simulink model "EKF_sim"  (R2020a)
settings: Solver=VariableStepAuto  StartTime=0.0  StopTime=257  RelTol=1e-3
values from neighbouring files (symbols this model uses):
  acc_variance = 4.8e-2    (= 0.048)    [init.m]
  bias_acc_variance = 4e-14    [init.m]
  bias_gyro_variance = 4e-14    [init.m]
  Delta2 = [260.168 -23.8158 1.64305]    [init.m]
  DT = EKF_DT    (= 0.01)    [init.m]
  EKF_DT = 0.01    [init.m]
  g = 9.81    [init.m]
  GPS_variance = 5    [init.m]
  gyro_variance = 4.8e-6    (= 4.8e-06)    [init.m]
  h0 = 38.8887000000000000    (= 38.8887)    [init.m]
  head_variance = 5e-2    (= 0.05)    [init.m]
  init_time = 4    [init.m]
  lambda_xa = 1e-4    (= 0.0001)    [init.m]
  lambda_xg = 1e-3    (= 0.001)    [init.m]
  lat0 = 36.7144590750000006    (= 36.714459075)    [init.m]
  lon0 = -4.4789588283333330    (= -4.47895882833)    [init.m]
  SHOE_buffer_N = 100    [init.m]
  SHOE_threshold = 2000    [init.m]
  t1_end = 100    [init.m]
  t1_start = 90    [init.m]
  t2_end = 193    [init.m]
  t2_start = 183    [init.m]
  t3_end = 213    [init.m]
  t3_start = 203    [init.m]
  t4_end = 244    [init.m]
  t4_start = 237    [init.m]
  type_of_GPS = 1    [init.m]
  vel_variance = 1e-2    (= 0.01)    [init.m]
  zero_vel_period = 0.1    [init.m]
(part 3 of 5)

== matlab function EKF_sim/EKF_nb/System Update/Flag Update/flag_updates ==
  data: time input; flag_updates_vector output size=1 3; SHOE_idx output; SHOE_buffer output; clk_zero_vel input; gyro input; acc input; pos_GPS input; hea_GPS input; SHOE_idx_prec input; SHOE_buffer_prec input; GPS_prec input; g parameter; GPS output; acc_variance parameter; gyro_variance parameter; SHOE_threshold parameter; SHOE_buffer_N parameter; t1_start parameter; t1_end parameter; t2_start parameter; t2_end parameter; t3_start parameter; t3_end parameter; ris output; t4_start parameter; t4_end parameter
% --------------------        flag_updates          -------------------- %
%{
% This function generate a flag vector containing informations of updates 
% for the correction step. There are three types of updates:

%  1. Zero Velocity constraints: we assume the vehicle moves only along its
%     x body axis direction, so the velocity in y and z axis are assumed to
%     be equal to zero.
%     The frequency of this update is based on signal 'clk_zero_vel', based
%     on 'zero_vel_period' parameter.
  
%  2. No-accelerating mode: when we detect a very low acceleration of the
%     vehicle, we can assume the accelerometer measures the gravity vector.
%     In this case we can update roll and pitch angles. SHOE algorithm is
%     used to detect a no-accelerating situation. (see [23] I. Skog et al., 
%     “Zero-Velocity Detection An Algorithm Evaluation,” IEEE Transactions 
%     on Biomedical Engineering, vol.57, no.11, pp.2657-2666, November
%     2010.)

%  3. Position and Heading updates: when a new value from GPS is detected,
%     position and heading is updated.

% In order to evaluate the EKF with GPS outages, we can block position and
% headings correction forced the corresponding flag to zero. This happens 
% in time intervals defined by the parameters t*_start and t*_end.

% Input:
%   time             : simulation time
%   clk_zero_vel     : clock of zero velocity constraints update
%   gyro             : [3x1] gyroscope measurement
%   acc              : [3x1] accelerometer measurement
%   pos_GPS          : [3x1] GPS data in NED
%   hea_GPS          : [1] Heading value from GPS data
%   SHOE_idx_prec    : previous buffer index for computation of SHOE algorithm
%   SHOE_buffer_prec : previous buffer for computation of SHOE algorithm
%   GPS_prec         : [4x1] previous data from GPS
%   g                : gravity acceleration
%   acc_variance     : Accelerometer Variance
%   gyro_variance    : Gyroscope Variance
%   SHOE_threshold   : Threshold for SHOE algorithm
%   SHOE_buffer_N    : Dimension of buffer for SHOE algorithm
%   t*_start         : start time i for GPS outage
%   t*_end           : end time i for GPS outage

% Output:
%   flag_updates_vector : [3x1] flag vector for new updates
%   SHOE_idx            : buffer index for computation of SHOE algorithm
%   SHOE_buffer         : buffer for computation of SHOE algorithm
%   GPS                 : [4x1] data from GPS
%   ris                 : Resultimg value of SHOE algorithm 
%}
%%
function [flag_updates_vector, SHOE_idx, SHOE_buffer, GPS,ris]  = flag_updates(time,clk_zero_vel, gyro, acc, pos_GPS, hea_GPS,...
                                                                         SHOE_idx_prec, SHOE_buffer_prec, GPS_prec, ...
                                                                         g, acc_variance, gyro_variance, SHOE_threshold, SHOE_buffer_N,...
                                                                         t1_start,t1_end,t2_start,t2_end,t3_start,t3_end,t4_start,t4_end)
    flag_updates_vector = zeros(1,3);
    
    %Dynamical constraints update (zero velocity)
    if clk_zero_vel == 1
        flag_updates_vector(1) = 1;
    end
    
    %Roll and Pitch Updates
    [SHOE_buffer, SHOE_idx, SHOE_flag,ris] = SHOE_detector(gyro, acc, SHOE_buffer_prec, SHOE_idx_prec, ...
                                                            SHOE_buffer_N, acc_variance, gyro_variance, SHOE_threshold, g); 
    if SHOE_flag == 1
        flag_updates_vector(2) = 1;
    end

    %Position and Heading Updates
    GPS = [pos_GPS(1), pos_GPS(2), pos_GPS(3), hea_GPS]';

    if ~isequal(GPS,GPS_prec)
        flag_updates_vector(3) = 1;
    end
    
    %Forced GPS outages
    if time > t1_start && time < t1_end
        flag_updates_vector(3) = 0;
    end
    if time > t2_start && time < t2_end
        flag_updates_vector(3) = 0;
    end
    if time > t3_start && time < t3_end
        flag_updates_vector(3) = 0;
    end
    if time > t4_start && time < t4_end
        flag_updates_vector(3) = 0;
    end
end

%% SHOE detector (ref.[23])
% This function detects if the acceleration of the vehicle is nearly zero.
% In that case we use the accelerometer measurements to estimates the 
% gravity vector in body frame and use it to update roll and pitch.
% For this purpose the mean of the last N measurements of accelerometer are
% compared to the gravity vector (magnitide and direction) and we use 
% gyroscope measurement to check if the vehicle is rotating. The resulting
% value stored in [ris] is compared with the SHOE Threshold.

function [SHOE_buffer, SHOE_idx, SHOE_flag,ris] = SHOE_detector(gyro, acc, SHOE_buffer, SHOE_idx, ...
                                                            SHOE_buffer_N, acc_variance, gyro_variance, SHOE_threshold, g) 
    %Buffer update with new measurement
    SHOE_buffer(SHOE_idx,:) = [acc(1), acc(2), acc(3), gyro(1), gyro(2), gyro(3)];
    SHOE_idx = SHOE_idx + 1;
    if SHOE_idx > SHOE_buffer_N
        SHOE_idx = 1;
    end

    %Detector Algorithm
    ya_n = [0 0 0];
    for i = 1:SHOE_buffer_N
        ya_n = ya_n + SHOE_buffer(i,1:3);	
    end
    ya_n = ya_n/SHOE_buffer_N;
    
    %calculate resulting maen value
    ris = 0; 
    for i = 1:SHOE_buffer_N
        ris = ris + (1/(acc_variance))*((norm(SHOE_buffer(i,1:3) - g*ya_n/norm(ya_n)))^2) + ...
                  + (1/(gyro_variance))*((norm(SHOE_buffer(i,4:6)))^2);
    end
    ris = ris/SHOE_buffer_N;
    
    if ris < SHOE_threshold
        SHOE_flag = 1;
    else 
        SHOE_flag = 0;
    end
end

%% %%%%%%%%%%%%%%%%%%%%%%%%%%%%%%%%%%%%%%%%%%%%%%%%%%%%%%%%%%%%%%%%%%%%%%%
     %%%%%%%%% Direct EKF for 6D Pose,  Marco Borraccino %%%%%%%%%%
     %%%%%%%%%   SGN Project, University of Pisa, 2021   %%%%%%%%%%
%%%%%%%%%%%%%%%%%%%%%%%%%%%%%%%%%%%%%%%%%%%%%%%%%%%%%%%%%%%%%%%%%%%%%%%%%%

== matlab function EKF_sim/EKF_nb/System Update/correction_step ==
  data: x_k_1 input; x_k output; P_k_1 input; e input size=9 1; H input size=9 16; R_k input size=9 9; P_k output; flag_init input
% --------------------         correction           -------------------- %
%{
% This function computes the correction step of the Kalman Filter. When new
% updates are avaiable, the Kalman Gain is updated and the vector state and
% matrix P too.

% Input:
%     x_k_1     : [16x1] state vector before correction step
%     P_k_1     : [16x16] matrix P before correction step
%     e         : [] Error between current measure and predicted measure
%     H         : [] Jacobian of prediction model measurement with respect 
%                 to state x
%     R_k       : [] Measurement Noise Covariance Matrix at time k
%     flag_init : flag for initialization task

% Output:
%     x_k       : [16x1] state vector after correction step
%     P_k       : [16x16] matrix P after correction step

% The formulas are?
%     S_k = H*P_k_1*H' + R_k;
%     K_k = P_k_1*H'*(inv(S_k));
%     P_k = (eye(16)-(K_k*H))*P_k_1;         
%     x_k = x_k_1 + K_k * e;
%}
%%
function [x_k, P_k] = correction(x_k_1, P_k_1, ...
                                 e, H, R_k, flag_init)
     x_k = zeros(16,1);
     P_k = zeros(16,16);
     
     if flag_init ~= -1
                
          S_k = H*P_k_1*H' + R_k;
          K_k = P_k_1*H'*(inv(S_k));

          P_k = (eye(16)-(K_k*H))*P_k_1;         
          x_k = x_k_1 + K_k * e;
     end
end

%% %%%%%%%%%%%%%%%%%%%%%%%%%%%%%%%%%%%%%%%%%%%%%%%%%%%%%%%%%%%%%%%%%%%%%%%
     %%%%%%%%% Direct EKF for 6D Pose,  Marco Borraccino %%%%%%%%%%
     %%%%%%%%%   SGN Project, University of Pisa, 2021   %%%%%%%%%%
%%%%%%%%%%%%%%%%%%%%%%%%%%%%%%%%%%%%%%%%%%%%%%%%%%%%%%%%%%%%%%%%%%%%%%%%%%

== matlab function EKF_sim/EKF_nb/System Update/virtual ==
  data: x_k input; R_ input; e output size=9 1; H output size=9 16; R_k output size=9 9; flag_updates_vector input; acc input; pos_GPS input; hea_GPS input; g parameter
% --------------------          virtual            -------------------- %
%{
% This function check the flag_updates_vector and produces the terms 'e',
% 'H' and 'R' based on it. When a flag update is set to zero by the
% previous function 'virtual', the dimensions of vector 'e' and matrices 
% 'H' and 'R' change to avoid wrong correction.
% There are three types of updates:

%  1. Zero Velocity constraints: we assume the vehicle moves only along its
%     x body axis direction, so the velocity in y and z axis are assumed to
%     be equal to zero.

%  2. No-accelerating mode: when we detect a very low acceleration of the
%     vehicle, we can assume the accelerometer measures the gravity vector.
%     In this case we can update roll and pitch angles.

%  3. Position and Heading updates: when a new value from GPS is detected,
%     position and heading is updated.

% For more deatils about matrix 'H' and the change of dimension, see file
% 'calcolo_matrice_H' and 'cutter_matrix'.

% Input:
%     x_k                 : [16x1] state vector before correction step
%     R_                  : [9x9] Measurement Noise Covariance Matrix
%     flag_updates_vector : [3x1] flag vector for new updates
%     acc                 : [3x1] Accelerometer Measurement
%     pos_GPS             : [3x1] GPS data in NED
%     hea_GPS             : [1] Heading value from GPS data
%     g                   : gravity acceleration

% Output:
%     e         : [] Error between current measure and predicted measure
%     H         : [] Jacobian of prediction model measurement with respect  
%                 to state x
%     R_k       : [] Measurement Noise Covariance Matrix at time k
%}
%%
function [e, H, R_k] = virtual(x_k, R_, flag_updates_vector, acc, pos_GPS, hea_GPS, g)

    e = zeros(9,1);
    h = zeros(9,1);
    z = zeros(9,1);
    H = zeros(9,16);
    q = x_k(1:4);
    
    %Dynamical constraints update (zero velocity)
    if  flag_updates_vector(1) == 1
        %hv0 = zeros(3,1);
        v  = x_k(11:13);
        Rnb = fromq2rot(q(1),q(2),q(3),q(4));
        hv0 = Rnb'*v;
        
        %z = z + [0       0    0 0 0 0 0 0 0]';
        h = h + [hv0(2) hv0(3) 0 0 0 0 0 0 0]';
        
        [H(1,:), H(2,:)]= calcolo_Hv0(q(1),q(2),q(3),q(4),v(1),v(2),v(3));
    end
    
    %Roll and Pitch Updates    
    if flag_updates_vector(2) == 1
        %hg = zeros(3,1);
        Rnb = fromq2rot(q(1),q(2),q(3),q(4));
        hg = Rnb'*[0 0 -g]';
        
        z = z + [0 0 acc(1) acc(2) acc(3) 0 0 0 0]';
        h = h + [0 0  hg(1)  hg(2)  hg(3) 0 0 0 0]';
        
        [H(3,:), H(4,:), H(5,:)]= calcolo_Hg(q(1),q(2),q(3),q(4),g);

    end
    
    %Position and Heading Updates
    if flag_updates_vector(3) == 1
        
        r = x_k(8:10);
        htheta = atan2(2*(q(2)*q(3)-q(1)*q(4)), 1-2*(q(3)^2+q(4)^2));
        
        z = z + [0 0 0 0 0 pos_GPS(1) pos_GPS(2) pos_GPS(3) hea_GPS]';
        h = h + [0 0 0 0 0    r(1)       r(2)       r(3)    htheta ]';
 
        H(6,:) = [0, 0, 0, 0, 0, 0, 0, 1, 0, 0, 0, 0, 0, 0, 0, 0];
        H(7,:) = [0, 0, 0, 0, 0, 0, 0, 0, 1, 0, 0, 0, 0, 0, 0, 0];
        H(8,:) = [0, 0, 0, 0, 0, 0, 0, 0, 0, 1, 0, 0, 0, 0, 0, 0];
        H(9,:)= calcolo_Htheta(q(1),q(2),q(3),q(4));  
    end
    e = z - h;
    coder.extrinsic('wrapToPi');
    if e(9)> pi
        e(9) = wrapToPi(e(9));
    end
    
    %After the generation of 'e', 'H' and 'R', we eliminate row and columns
    %of them if they are not used. The resultanting scaled vector and 
    %matrix are used in the next correction step function.
    R=R_;
    i=0;
    if  flag_updates_vector(1) == 0
        H(1-i,:) = [];
        e(1-i) = [];
        R(1-i,:) = [];
        R(:,1-i) = [];
        i=i+1;
        H(2-i,:) = [];
        e(2-i) = [];
        R(2-i,:) = [];
        R(:,2-i) = [];
        i=i+1;
    end
    if  flag_updates_vector(2) == 0
        H(3-i,:) = [];
        e(3-i) = [];
        R(3-i,:) = [];
        R(:,3-i) = [];
        i=i+1;
        H(4-i,:) = [];
        e(4-i) = [];
        R(4-i,:) = [];
        R(:,4-i) = [];
        i=i+1;
        H(5-i,:) = [];
        e(5-i) = [];
        R(5-i,:) = [];
        R(:,5-i) = [];
        i=i+1;
    end
    if  flag_updates_vector(3) == 0
        H(6-i,:) = [];
        e(6-i) = [];
        R(6-i,:) = [];
        R(:,6-i) = [];
        i=i+1;
        H(7-i,:) = [];
        e(7-i) = [];
        R(7-i,:) = [];
        R(:,7-i) = [];
        i=i+1;
        H(8-i,:) = [];
        e(8-i) = [];
        R(8-i,:) = [];
        R(:,8-i) = [];
        i=i+1;
        H(9-i,:) = [];
        e(9-i) = [];
        R(9-i,:) = [];
        R(:,9-i) = [];
    end
    R_k=R;
end

%% Auxiliary Functions
% This function computes the rotation matrix from quaternion
function rot = fromq2rot(q1,q2,q3,q4)
    rot = [q1^2+q2^2-q3^2-q4^2, 2*(q2*q3-q1*q4), 2*(q1*q3+q2*q4); ...
           2*(q2*q3+q1*q4), q1^2-q2^2+q3^2-q4^2, 2*(q3*q4-q1*q2); ...
           2*(q2*q4-q1*q3), 2*(q1*q2+q3*q4), q1^2-q2^2-q3^2+q4^2];
end
%%
% These functions calculate the H matrix elements
% See 'calcolo_matrice_H_nb.m' for the symbolic calculation used
function [Hv01 , Hv02] = calcolo_Hv0(q1,q2,q3,q4,vx,vy,vz)  
    Hv01 = [ 2*q1*vy - 2*q4*vx + 2*q2*vz, 2*q3*vx - 2*q2*vy + 2*q1*vz, 2*q2*vx + 2*q3*vy + 2*q4*vz, 2*q3*vz - 2*q4*vy - 2*q1*vx, 0, 0, 0, 0, 0, 0, 2*q2*q3 - 2*q1*q4, q1^2 - q2^2 + q3^2 - q4^2, 2*q1*q2 + 2*q3*q4, 0, 0, 0];
    Hv02 = [ 2*q3*vx - 2*q2*vy + 2*q1*vz, 2*q4*vx - 2*q1*vy - 2*q2*vz, 2*q1*vx + 2*q4*vy - 2*q3*vz, 2*q2*vx + 2*q3*vy + 2*q4*vz, 0, 0, 0, 0, 0, 0, 2*q1*q3 + 2*q2*q4, 2*q3*q4 - 2*q1*q2, q1^2 - q2^2 - q3^2 + q4^2, 0, 0, 0];
end
function [Hg1 , Hg2, Hg3] = calcolo_Hg(q1,q2,q3,q4,g)
    Hg1 = [  2*g*q3, -2*g*q4,  2*g*q1, -2*g*q2, 0, 0, 0, 0, 0, 0, 0, 0, 0, 0, 0, 0];
    Hg2 = [ -2*g*q2, -2*g*q1, -2*g*q4, -2*g*q3, 0, 0, 0, 0, 0, 0, 0, 0, 0, 0, 0, 0];
    Hg3 = [ -2*g*q1,  2*g*q2,  2*g*q3, -2*g*q4, 0, 0, 0, 0, 0, 0, 0, 0, 0, 0, 0, 0];
end
function Htheta= calcolo_Htheta(q1,q2,q3,q4)
    Htheta = [ (2*q4*(2*q3^2 + 2*q4^2 - 1))/((2*q3^2 + 2*q4^2 - 1)^2 + (2*q1*q4 - 2*q2*q3)^2), -(2*q3*(2*q3^2 + 2*q4^2 - 1))/((2*q3^2 + 2*q4^2 - 1)^2 + (2*q1*q4 - 2*q2*q3)^2), -(((2*q2)/(2*q3^2 + 2*q4^2 - 1) + (4*q3*(2*q1*q4 - 2*q2*q3))/(2*q3^2 + 2*q4^2 - 1)^2)*(2*q3^2 + 2*q4^2 - 1)^2)/((2*q3^2 + 2*q4^2 - 1)^2 + (2*q1*q4 - 2*q2*q3)^2), (((2*q1)/(2*q3^2 + 2*q4^2 - 1) - (4*q4*(2*q1*q4 - 2*q2*q3))/(2*q3^2 + 2*q4^2 - 1)^2)*(2*q3^2 + 2*q4^2 - 1)^2)/((2*q3^2 + 2*q4^2 - 1)^2 + (2*q1*q4 - 2*q2*q3)^2), 0, 0, 0, 0, 0, 0, 0, 0, 0, 0, 0, 0];
end

%% %%%%%%%%%%%%%%%%%%%%%%%%%%%%%%%%%%%%%%%%%%%%%%%%%%%%%%%%%%%%%%%%%%%%%%%
     %%%%%%%%% Direct EKF for 6D Pose,  Marco Borraccino %%%%%%%%%%
     %%%%%%%%%   SGN Project, University of Pisa, 2021   %%%%%%%%%%
%%%%%%%%%%%%%%%%%%%%%%%%%%%%%%%%%%%%%%%%%%%%%%%%%%%%%%%%%%%%%%%%%%%%%%%%%%

== matlab function EKF_sim/MATLAB Function1 ==
  data: or_rad output; u input
% --------------------          quat2ypr            -------------------- %
%{
% This function transform attitude quaternion in Euler angles
%}

function or_rad  = quat2ypr(u)
q = quaternion([u(1) u(2) u(3) u(4)]);
or_rad = [0,0,0]';
or_rad = (euler(q,'zyx','frame'))';
end


%% %%%%%%%%%%%%%%%%%%%%%%%%%%%%%%%%%%%%%%%%%%%%%%%%%%%%%%%%%%%%%%%%%%%%%%%
     %%%%%%%%% Direct EKF for 6D Pose,  Marco Borraccino %%%%%%%%%%
     %%%%%%%%%   SGN Project, University of Pisa, 2021   %%%%%%%%%%
%%%%%%%%%%%%%%%%%%%%%%%%%%%%%%%%%%%%%%%%%%%%%%%%%%%%%%%%%%%%%%%%%%%%%%%%%%%

== matlab function EKF_sim/MATLAB Function4 ==
  data: GPS input; GPS_NED output; lon0 parameter; lat0 parameter; h0 parameter
% --------------------          ECEF2NED            -------------------- %
%{
% This function transform the GPS data from ECEF to NED reference system.
% 'geodetic2ned' function is used with 'wgs84' Earth model.

% Input:
%     GPS         : GPS data [3x1] lat-lon-h [degree,degree,m]
%     lon0        : Origin Longitude of NED
%     lat0        : Origin Latitude of NED
%     h0          : Origin Height of NED

% Output:
%     GPS_NED     : GPS data [3x1] in NED North-East-Down [m]

%}
%%
function GPS_NED = ECEF2NED(GPS,lon0,lat0,h0)
    GPS_NED = [0 0 0]';
    coder.extrinsic('evalin', 'wgs84Ellipsoid', 'geodetic2ned');
    [GPS_NED(1),GPS_NED(2),GPS_NED(3)]= geodetic2ned(GPS(1), GPS(2), GPS(3),...
                                                     lat0, lon0, h0, wgs84Ellipsoid,'degree');
end

%% %%%%%%%%%%%%%%%%%%%%%%%%%%%%%%%%%%%%%%%%%%%%%%%%%%%%%%%%%%%%%%%%%%%%%%%
     %%%%%%%%% Direct EKF for 6D Pose,  Marco Borraccino %%%%%%%%%%
     %%%%%%%%%   SGN Project, University of Pisa, 2021   %%%%%%%%%%
%%%%%%%%%%%%%%%%%%%%%%%%%%%%%%%%%%%%%%%%%%%%%%%%%%%%%%%%%%%%%%%%%%%%%%%%%%

== matlab function EKF_sim/MATLAB Function5 ==
  data: u input; y output
function y = wrap2pi(u)
    y = 0;
    coder.extrinsic('wrapToPi');

    y = wrapToPi(u);
end

== matlab function EKF_sim/MATLAB Function7 ==
  data: u input; dev_x output; dev_y output; dev_z output
function [dev_x, dev_y, dev_z] = fcn(u)

    dev_x = sqrt(u(11,11));
    dev_y = sqrt(u(12,12));
    dev_z = sqrt(u(13,13));

end

== matlab function EKF_sim/EKF_bias/MATLAB Function ==
  data: GPS input; GPS_NED output; lon0 parameter; lat0 parameter; h0 parameter
% --------------------          ECEF2NED            -------------------- %
%{
% This function transform the GPS data from ECEF to NED reference system.
% 'geodetic2ned' function is used with 'wgs84' Earth model.

% Input:
%     GPS         : GPS data [3x1] lat-lon-h [degree,degree,m]
%     lon0        : Origin Longitude of NED
%     lat0        : Origin Latitude of NED
%     h0          : Origin Height of NED

% Output:
%     GPS_NED     : GPS data [3x1] in NED North-East-Down [m]

%}
%%
function GPS_NED = ECEF2NED(GPS,lon0,lat0,h0)
    GPS_NED = [0 0 0];
    coder.extrinsic('evalin', 'wgs84Ellipsoid', 'geodetic2ned');
    [GPS_NED(1),GPS_NED(2),GPS_NED(3)]= geodetic2ned(GPS(1), GPS(2), GPS(3),...
                                                     lat0, lon0, h0, wgs84Ellipsoid,'degree');
end

%% %%%%%%%%%%%%%%%%%%%%%%%%%%%%%%%%%%%%%%%%%%%%%%%%%%%%%%%%%%%%%%%%%%%%%%%
     %%%%%%%%% Direct EKF for 6D Pose,  Marco Borraccino %%%%%%%%%%
     %%%%%%%%%   SGN Project, University of Pisa, 2021   %%%%%%%%%%
%%%%%%%%%%%%%%%%%%%%%%%%%%%%%%%%%%%%%%%%%%%%%%%%%%%%%%%%%%%%%%%%%%%%%%%%%%

== matlab function EKF_sim/EKF_bias/Initialization task/Initialization task ==
  data: flag_init input; flag_init output; acc input; gyro input; head input; x0 output; P0 output; buffer input; buffer output; buffer_idx input; buffer_idx output; init_time parameter; acc_variance parameter; Delta2 parameter
% --------------------          EKF_init            -------------------- %
%{
% This function computes the initialization task at the start of the
% simulation. The initial attitude and gyroscope bias is calculated from 
% the mean value of the measurement in period [0,init_time]. 
% The matrix P is also initialized with a estimated attitude 
% covariance, see [27] (R. Munguia and A. Grau, "A Practical Method for 
% Implementing an Attitude and Heading Reference System," International 
% Journal of Advanced Robotic Systems, vol. 11, 2014) for more details.

% Input:
%     flag_init    : flag for initialization task
%     acc          : accelerometer measurement
%     gyro         : gyroscope measurement
%     head         : Heading measurement from GPS
%     Delta2       : NED reference system Offset
%     buffer       : buffer for calculate the initial mean valus 
%     buffer_idx   : index of buffer for calculate the initial mean value
%     init_time    : Initial period of time for initialization task 
%     acc_variance : Accelerometer Variance

% Output:
%     flag_init    : flag for initialization task
%     x0           : initial vector state
%     P0           : initial matrix P
%     buffer       : buffer for calculate the initial mean valus 
%     buffer_idx   : index of buffer for calculate the initial mean value
%}
%%
function [flag_init, x0, P0,buffer,buffer_idx] = EKF_init(flag_init, acc,gyro,head,buffer,buffer_idx, init_time,acc_variance, Delta2)
    x0 = zeros(22,1);
    P0 = zeros(22,22);
    
    %fill the buffer with initial sensors measurements
    if flag_init == -1
        buffer(buffer_idx,1:3) = -acc;
        buffer(buffer_idx,4:6) = gyro;
        buffer(buffer_idx,7) = head;
        buffer_idx = buffer_idx + 1;
    end

    if buffer_idx == 100*init_time && flag_init == -1 %..after [init_time]
        
        %calculate initial value of state variable and matrix P
        g0          = mean(buffer(:,1:3));  
        bgyro_init  = mean(buffer(:,4:6));
        roll_init   = atan2(g0(2),g0(3));
        pitch_init  = atan2(-g0(1),(g0(2)^2+g0(3)^2)^0.5);
        yaw_init    = pi/2;
%        yaw_init    = mean(buffer(:,7));
        
        q = new_q(yaw_init,pitch_init,roll_init);
        x0 = [  q(1)              q(2)            q(3)            q(4)    ...
                0                 0               0                       ...
                bgyro_init(1)     bgyro_init(2)   bgyro_init(3)           ...
                Delta2(2)         Delta2(1)       -Delta2(3)              ...
                0                 0               0                       ...
                0                 0               0                       ...
                0                 0               0                       ]';
        Pq = Pq_init_calculation(roll_init,pitch_init,yaw_init,acc_variance,init_time); 
        P0 = blkdiag(Pq, diag([ 4.8e-6  4.8e-6  4.8e-6          ...
                                1e-7    1e-7    1e-7            ...
                                1       1       1               ...
                                0.1     0.1     0.1             ...
                                4.8e-2  4.8e-2  4.8e-2          ...
                                1e-3    1e-3    1e-3            ]));
        flag_init = 1;
    end
end

%% Auxiliary Functions
% This function calculate the initial Pq0, in the same manner as [27].
% % See 'calcolo_matrice_Pq0.m' for the symbolic calculation used.
function Pq = Pq_init_calculation(roll,pitch,yaw,acc_variance,init_time)
    P_ = eye(3)* acc_variance/(init_time*100);
    dq= [                                                                                                                                                                                                                                -(cos(pitch)*sin(roll) + cos(yaw)*sin(roll) - cos(roll)*sin(pitch)*sin(yaw))/(2*(cos(pitch)*cos(roll) + cos(pitch)*cos(yaw) + cos(roll)*cos(yaw) + sin(pitch)*sin(roll)*sin(yaw) + 1)^(1/2)),                                                                                                                                                                                                                        -(cos(roll)*sin(pitch) + cos(yaw)*sin(pitch) - cos(pitch)*sin(roll)*sin(yaw))/(2*(cos(pitch)*cos(roll) + cos(pitch)*cos(yaw) + cos(roll)*cos(yaw) + sin(pitch)*sin(roll)*sin(yaw) + 1)^(1/2)),                                                                                                                                                                                                                                -(cos(pitch)*sin(yaw) + cos(roll)*sin(yaw) - cos(yaw)*sin(pitch)*sin(roll))/(2*(cos(pitch)*cos(roll) + cos(pitch)*cos(yaw) + cos(roll)*cos(yaw) + sin(pitch)*sin(roll)*sin(yaw) + 1)^(1/2));
                   - cos(roll)*cos(yaw) - (cos(pitch)*cos(roll))/(4*(cos(pitch)*cos(roll) + cos(pitch)*cos(yaw) + cos(roll)*cos(yaw) + sin(pitch)*sin(roll)*sin(yaw) + 1)^(1/2)) - sin(pitch)*sin(roll)*sin(yaw) - (cos(pitch)*sin(roll)*(cos(pitch)*sin(roll) + cos(yaw)*sin(roll) - cos(roll)*sin(pitch)*sin(yaw)))/(8*(cos(pitch)*cos(roll) + cos(pitch)*cos(yaw) + cos(roll)*cos(yaw) + sin(pitch)*sin(roll)*sin(yaw) + 1)^(3/2)),                         (sin(pitch)*sin(roll))/(4*(cos(pitch)*cos(roll) + cos(pitch)*cos(yaw) + cos(roll)*cos(yaw) + sin(pitch)*sin(roll)*sin(yaw) + 1)^(1/2)) + cos(pitch)*cos(roll)*sin(yaw) - (cos(pitch)*sin(roll)*(cos(roll)*sin(pitch) + cos(yaw)*sin(pitch) - cos(pitch)*sin(roll)*sin(yaw)))/(8*(cos(pitch)*cos(roll) + cos(pitch)*cos(yaw) + cos(roll)*cos(yaw) + sin(pitch)*sin(roll)*sin(yaw) + 1)^(3/2)),                                                                                                                                                     sin(roll)*sin(yaw) + cos(roll)*cos(yaw)*sin(pitch) - (cos(pitch)*sin(roll)*(cos(pitch)*sin(yaw) + cos(roll)*sin(yaw) - cos(yaw)*sin(pitch)*sin(roll)))/(8*(cos(pitch)*cos(roll) + cos(pitch)*cos(yaw) + cos(roll)*cos(yaw) + sin(pitch)*sin(roll)*sin(yaw) + 1)^(3/2));
          - (cos(roll)*sin(yaw) - cos(yaw)*sin(pitch)*sin(roll))/(4*(cos(pitch)*cos(roll) + cos(pitch)*cos(yaw) + cos(roll)*cos(yaw) + sin(pitch)*sin(roll)*sin(yaw) + 1)^(1/2)) - ((sin(roll)*sin(yaw) + cos(roll)*cos(yaw)*sin(pitch))*(cos(pitch)*sin(roll) + cos(yaw)*sin(roll) - cos(roll)*sin(pitch)*sin(yaw)))/(8*(cos(pitch)*cos(roll) + cos(pitch)*cos(yaw) + cos(roll)*cos(yaw) + sin(pitch)*sin(roll)*sin(yaw) + 1)^(3/2)), - cos(pitch) - ((sin(roll)*sin(yaw) + cos(roll)*cos(yaw)*sin(pitch))*(cos(roll)*sin(pitch) + cos(yaw)*sin(pitch) - cos(pitch)*sin(roll)*sin(yaw)))/(8*(cos(pitch)*cos(roll) + cos(pitch)*cos(yaw) + cos(roll)*cos(yaw) + sin(pitch)*sin(roll)*sin(yaw) + 1)^(3/2)) - (cos(pitch)*cos(roll)*cos(yaw))/(4*(cos(pitch)*cos(roll) + cos(pitch)*cos(yaw) + cos(roll)*cos(yaw) + sin(pitch)*sin(roll)*sin(yaw) + 1)^(1/2)), - (cos(yaw)*sin(roll) - cos(roll)*sin(pitch)*sin(yaw))/(4*(cos(pitch)*cos(roll) + cos(pitch)*cos(yaw) + cos(roll)*cos(yaw) + sin(pitch)*sin(roll)*sin(yaw) + 1)^(1/2)) - ((sin(roll)*sin(yaw) + cos(roll)*cos(yaw)*sin(pitch))*(cos(pitch)*sin(yaw) + cos(roll)*sin(yaw) - cos(yaw)*sin(pitch)*sin(roll)))/(8*(cos(pitch)*cos(roll) + cos(pitch)*cos(yaw) + cos(roll)*cos(yaw) + sin(pitch)*sin(roll)*sin(yaw) + 1)^(3/2));
                                                                                                                                                              sin(roll)*sin(yaw) + cos(roll)*cos(yaw)*sin(pitch) - (cos(pitch)*sin(yaw)*(cos(pitch)*sin(roll) + cos(yaw)*sin(roll) - cos(roll)*sin(pitch)*sin(yaw)))/(8*(cos(pitch)*cos(roll) + cos(pitch)*cos(yaw) + cos(roll)*cos(yaw) + sin(pitch)*sin(roll)*sin(yaw) + 1)^(3/2)),                           (sin(pitch)*sin(yaw))/(4*(cos(pitch)*cos(roll) + cos(pitch)*cos(yaw) + cos(roll)*cos(yaw) + sin(pitch)*sin(roll)*sin(yaw) + 1)^(1/2)) + cos(pitch)*cos(yaw)*sin(roll) - (cos(pitch)*sin(yaw)*(cos(roll)*sin(pitch) + cos(yaw)*sin(pitch) - cos(pitch)*sin(roll)*sin(yaw)))/(8*(cos(pitch)*cos(roll) + cos(pitch)*cos(yaw) + cos(roll)*cos(yaw) + sin(pitch)*sin(roll)*sin(yaw) + 1)^(3/2)),            - cos(roll)*cos(yaw) - (cos(pitch)*cos(yaw))/(4*(cos(pitch)*cos(roll) + cos(pitch)*cos(yaw) + cos(roll)*cos(yaw) + sin(pitch)*sin(roll)*sin(yaw) + 1)^(1/2)) - sin(pitch)*sin(roll)*sin(yaw) - (cos(pitch)*sin(yaw)*(cos(pitch)*sin(yaw) + cos(roll)*sin(yaw) - cos(yaw)*sin(pitch)*sin(roll)))/(8*(cos(pitch)*cos(roll) + cos(pitch)*cos(yaw) + cos(roll)*cos(yaw) + sin(pitch)*sin(roll)*sin(yaw) + 1)^(3/2))];
    Pq = dq*P_*dq';
end

% This function create a quaternion from Euler's angle [Yaw,Pitch,Roll]
function q = new_q(yaw,pitch,roll)
    q = zeros(1,4);
    q(1) = cos(roll/2) * cos(pitch/2) * cos(yaw/2) + sin(roll/2) * sin(pitch/2) * sin(yaw/2);
    q(2) = sin(roll/2) * cos(pitch/2) * cos(yaw/2) - cos(roll/2) * sin(pitch/2) * sin(yaw/2);
    q(3) = cos(roll/2) * sin(pitch/2) * cos(yaw/2) + sin(roll/2) * cos(pitch/2) * sin(yaw/2);
    q(4) = cos(roll/2) * cos(pitch/2) * sin(yaw/2) - sin(roll/2) * sin(pitch/2) * cos(yaw/2);  
end

%% %%%%%%%%%%%%%%%%%%%%%%%%%%%%%%%%%%%%%%%%%%%%%%%%%%%%%%%%%%%%%%%%%%%%%%%
     %%%%%%%%% Direct EKF for 6D Pose,  Marco Borraccino %%%%%%%%%%
     %%%%%%%%%   SGN Project, University of Pisa, 2021   %%%%%%%%%%
%%%%%%%%%%%%%%%%%%%%%%%%%%%%%%%%%%%%%%%%%%%%%%%%%%%%%%%%%%%%%%%%%%%%%%%%%%

== matlab function EKF_sim/EKF_bias/System Update/Flag Update/flag_updates ==
  data: time input; flag_updates_vector output size=1 3; SHOE_idx output; SHOE_buffer output; clk_zero_vel input; gyro input; acc input; pos_GPS input; hea_GPS input; SHOE_idx_prec input; SHOE_buffer_prec input; GPS_prec input; g parameter; GPS output; acc_variance parameter; gyro_variance parameter; SHOE_threshold parameter; SHOE_buffer_N parameter; t1_start parameter; t1_end parameter; t2_start parameter; t2_end parameter; t3_start parameter; t3_end parameter; ris output; t4_start parameter; t4_end parameter
% --------------------        flag_updates          -------------------- %
%{
% This function generate a flag vector containing informations of updates 
% for the correction step. There are three types of updates:

%  1. Zero Velocity constraints: we assume the vehicle moves only along its
%     x body axis direction, so the velocity in y and z axis are assumed to
%     be equal to zero.
%     The frequency of this update is based on signal 'clk_zero_vel', based
%     on 'zero_vel_period' parameter.
  
%  2. No-accelerating mode: when we detect a very low acceleration of the
%     vehicle, we can assume the accelerometer measures the gravity vector.
%     In this case we can update roll and pitch angles. SHOE algorithm is
%     used to detect a no-accelerating situation. (see [23] I. Skog et al., 
%     “Zero-Velocity Detection An Algorithm Evaluation,” IEEE Transactions 
%     on Biomedical Engineering, vol.57, no.11, pp.2657-2666, November
%     2010.)

%  3. Position and Heading updates: when a new value from GPS is detected,
%     position and heading is updated.

% In order to evaluate the EKF with GPS outages, we can block position and
% headings correction forced the corresponding flag to zero. This happens 
% in time intervals defined by the parameters t*_start and t*_end.

% Input:
%   time             : simulation time
%   clk_zero_vel     : clock of zero velocity constraints update
%   gyro             : [3x1] gyroscope measurement
%   acc              : [3x1] accelerometer measurement
%   pos_GPS          : [3x1] GPS data in NED
%   hea_GPS          : [1] Heading value from GPS data
%   SHOE_idx_prec    : previous buffer index for computation of SHOE algorithm
%   SHOE_buffer_prec : previous buffer for computation of SHOE algorithm
%   GPS_prec         : [4x1] previous data from GPS
%   g                : gravity acceleration
%   acc_variance     : Accelerometer Variance
%   gyro_variance    : Gyroscope Variance
%   SHOE_threshold   : Threshold for SHOE algorithm
%   SHOE_buffer_N    : Dimension of buffer for SHOE algorithm
%   t*_start         : start time i for GPS outage
%   t*_end           : end time i for GPS outage

% Output:
%   flag_updates_vector : [3x1] flag vector for new updates
%   SHOE_idx            : buffer index for computation of SHOE algorithm
%   SHOE_buffer         : buffer for computation of SHOE algorithm
%   GPS                 : [4x1] data from GPS
%   ris                 : Resultimg value of SHOE algorithm 
%}
%%
function [flag_updates_vector, SHOE_idx, SHOE_buffer, GPS,ris]  = flag_updates(time,clk_zero_vel, gyro, acc, pos_GPS, hea_GPS,...
                                                                         SHOE_idx_prec, SHOE_buffer_prec, GPS_prec, ...
                                                                         g, acc_variance, gyro_variance, SHOE_threshold, SHOE_buffer_N,...
                                                                         t1_start,t1_end,t2_start,t2_end,t3_start,t3_end,t4_start,t4_end)
    flag_updates_vector = zeros(1,3);
    
    %Dynamical constraints update (zero velocity)
    if clk_zero_vel == 1
        flag_updates_vector(1) = 1;
    end
    
    %Roll and Pitch Updates
    [SHOE_buffer, SHOE_idx, SHOE_flag,ris] = SHOE_detector(gyro, acc, SHOE_buffer_prec, SHOE_idx_prec, ...
                                                            SHOE_buffer_N, acc_variance, gyro_variance, SHOE_threshold, g); 
    if SHOE_flag == 1
        flag_updates_vector(2) = 1;
    end

    %Position and Heading Updates
    GPS = [pos_GPS(1), pos_GPS(2), pos_GPS(3), hea_GPS]';

    if ~isequal(GPS,GPS_prec)
        flag_updates_vector(3) = 1;
    end
    
    %Forced GPS outages
    if time > t1_start && time < t1_end
        flag_updates_vector(3) = 0;
    end
    if time > t2_start && time < t2_end
        flag_updates_vector(3) = 0;
    end
    if time > t3_start && time < t3_end
        flag_updates_vector(3) = 0;
    end
    if time > t4_start && time < t4_end
        flag_updates_vector(3) = 0;
    end
end

%% SHOE detector (ref.[23])
% This function detects if the acceleration of the vehicle is nearly zero.
% In that case we use the accelerometer measurements to estimates the 
% gravity vector in body frame and use it to update roll and pitch.
% For this purpose the mean of the last N measurements of accelerometer are
% compared to the gravity vector (magnitide and direction) and we use 
% gyroscope measurement to check if the vehicle is rotating. The resulting
% value stored in [ris] is compared with the SHOE Threshold.

function [SHOE_buffer, SHOE_idx, SHOE_flag,ris] = SHOE_detector(gyro, acc, SHOE_buffer, SHOE_idx, ...
                                                            SHOE_buffer_N, acc_variance, gyro_variance, SHOE_threshold, g) 
    %Buffer update with new measurement
    SHOE_buffer(SHOE_idx,:) = [acc(1), acc(2), acc(3), gyro(1), gyro(2), gyro(3)];
    SHOE_idx = SHOE_idx + 1;
    if SHOE_idx > SHOE_buffer_N
        SHOE_idx = 1;
    end

    %Detector Algorithm
    ya_n = [0 0 0];
    for i = 1:SHOE_buffer_N
        ya_n = ya_n + SHOE_buffer(i,1:3);	
    end
    ya_n = ya_n/SHOE_buffer_N;
    
    %calculate resulting maen value
    ris = 0; 
    for i = 1:SHOE_buffer_N
        ris = ris + (1/(acc_variance))*((norm(SHOE_buffer(i,1:3) - g*ya_n/norm(ya_n)))^2) + ...
                  + (1/(gyro_variance))*((norm(SHOE_buffer(i,4:6)))^2);
    end
    ris = ris/SHOE_buffer_N;
    
    if ris < SHOE_threshold
        SHOE_flag = 1;
    else 
        SHOE_flag = 0;
    end
end

%% %%%%%%%%%%%%%%%%%%%%%%%%%%%%%%%%%%%%%%%%%%%%%%%%%%%%%%%%%%%%%%%%%%%%%%%
     %%%%%%%%% Direct EKF for 6D Pose,  Marco Borraccino %%%%%%%%%%
     %%%%%%%%%   SGN Project, University of Pisa, 2021   %%%%%%%%%%
%%%%%%%%%%%%%%%%%%%%%%%%%%%%%%%%%%%%%%%%%%%%%%%%%%%%%%%%%%%%%%%%%%%%%%%%%%
